simulink model "Orifice_Test"  (R2013a)
settings: Solver=ode15s  StartTime=0.0  StopTime=10.0  RelTol=1e-3  AbsTol=1e-4
libraries: fl_lib x4, nesl_utility x3, Hydraulic_lib x1, sh_lib x1
Description:
  | Copyright 2013 The MathWorks, Inc.
settings Model: Creator=smiller  LastModifiedBy=smiller
settings OptimizationCC: ExpressionDepthLimit=2147483647

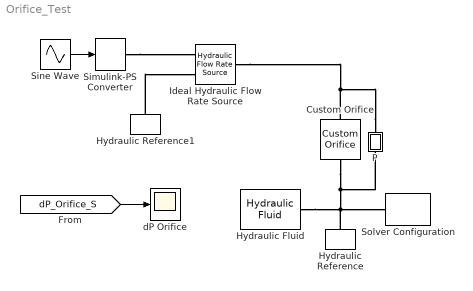
== system Orifice_Test ==
  Custom Orifice : Hydraulic_lib/Custom Orifice  area=1e-5 m^2  Cd=0.7  Recr=12  q_Log=off  p_Log=off  Re_Log=off  LocalVarNames=|q|p|Re  LocalVarDescs=|Volumetric flow rate|Pressure|Reynolds number  LocalVarLogging=[0 0 0]
  Hydraulic Fluid : sh_lib/Hydraulic Utilities/Hydraulic Fluid  DataSource=1  SelFluid=1  SysTemp=60 c  TrapAir=0.005  ViscDerFactor=1  LocalVarLogging=[]
  Hydraulic Reference : fl_lib/Hydraulic/Hydraulic Elements/Hydraulic Reference  q_Log=off  LocalVarNames=|q  LocalVarDescs=|q  LocalVarLogging=[]
  Hydraulic Reference1 : fl_lib/Hydraulic/Hydraulic Elements/Hydraulic Reference  q_Log=off  LocalVarNames=|q  LocalVarDescs=|q  LocalVarLogging=[]
  Ideal Hydraulic Flow Rate Source : fl_lib/Hydraulic/Hydraulic Sources/Hydraulic Flow Rate Source  q_Log=off  p_Log=off  LocalVarNames=|flow_rate|pr_differential|power  LocalVarDescs=|Flow rate through the source (m^3/s)|Pressure differential across the source (Pa)|Source power (W)  LocalVarLogging=[0 0 0]
  P : Subsystem
      mask Display: disp('P');
  Simulink-PS Converter : nesl_utility/Simulink-PS Converter  PhysicalDomain=network_engine_domain  SubClassName=ps_input  LeftPortType=input  RightPortType=output  PseudoPeriodic=off  Frequencies=[]  NoiseDistribution=none  NoiseParameters=[]  Unit=lpm  AffineConversion=off  InputFiltering=off  SimscapeFilterOrder=1  InputFilterTimeConstant=.001  UdotUserProvided=1
  Sine Wave : Sin  Bias=0.1  SampleTime=0
  Solver Configuration : nesl_utility/Solver Configuration  PhysicalDomain=network_engine_domain  SubClassName=solver  LeftPortType=input  RightPortType=generic  Accelerate=off  Tones=[]  Harmonics=[]  SimulateNoise=off  Profile=off  UseLocalSampling=off  EnableSwitchedLinearOptims=on  FrequencyDomain=off  UseCCode=off  UseNewInitialization=off  DoDC=off  ResidualTolerance=1e-9  UseLocalSolver=off  LocalSolverChoice=NE_BACKWARD_EULER_ADVANCER  LocalSolverSampleTime=.001  DoFixedCost=off  MaxNonlinIter=12  MaxModeIter=2  LinearAlgebra=Sparse  DelaysMemoryBudget=1024
  dP Orifice : Scope
      settings: YMin=-4000  YMax=6000  SaveName=dP_Orifice_DATA
  wires:
  Sine Wave/1 -> Simulink-PS Converter/1
  [dP_Orifice_S] -> dP Orifice/1
  connections:
  P/LConn1 -- Custom Orifice/LConn1 -- Ideal Hydraulic Flow Rate Source/LConn1
  P/RConn1 -- Custom Orifice/RConn1 -- Hydraulic Fluid/RConn1 -- Hydraulic Reference/LConn1 -- Solver Configuration/RConn1
  Simulink-PS Converter/RConn1 -- Ideal Hydraulic Flow Rate Source/RConn1
  Hydraulic Reference1/LConn1 -- Ideal Hydraulic Flow Rate Source/RConn2

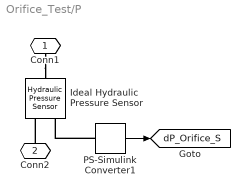
== system Orifice_Test/P ==
  Ideal Hydraulic Pressure Sensor : fl_lib/Hydraulic/Hydraulic Sensors/Hydraulic Pressure Sensor  q_Log=off  p_Log=off  LocalVarNames=|q|p  LocalVarDescs=|q|p  LocalVarLogging=[]
  PS-Simulink Converter1 : nesl_utility/PS-Simulink Converter  PhysicalDomain=network_engine_domain  SubClassName=ps_output  LeftPortType=input  RightPortType=output  PseudoPeriodic=off  Frequencies=[]  Unit=Pa  AffineConversion=off
  Conn1 : PMIOPort  Port=1  Side=Left
  Conn2 : PMIOPort  Port=2  Side=Right
  tag scope: dP_Orifice_S=global
  wires:
  PS-Simulink Converter1/1 -> [dP_Orifice_S]
  connections:
  PS-Simulink Converter1/LConn1 -- Ideal Hydraulic Pressure Sensor/RConn2
  Conn1/RConn1 -- Ideal Hydraulic Pressure Sensor/LConn1
  Conn2/RConn1 -- Ideal Hydraulic Pressure Sensor/RConn1
